simulink model "Sub_SC_G_based_221015"  (R2022b)
settings: Solver=VariableStepAuto  StartTime=0.0  StopTime=10.0  RelTol=1e-3
undefined symbols (not defined in the file or in its folder): R_bal, SC_rc, SC_rv
libraries: spsCurrentMeasurementLib x2, spsSeriesRLCBranchLib x2, spsSupercapacitorLib x1
settings Model: Creator=xuupp  LastModifiedBy=xuupp

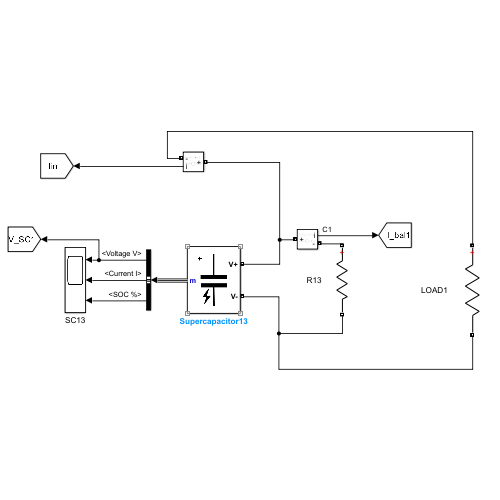
[thumbnail: Simulink's stored preview of the top-level diagram]
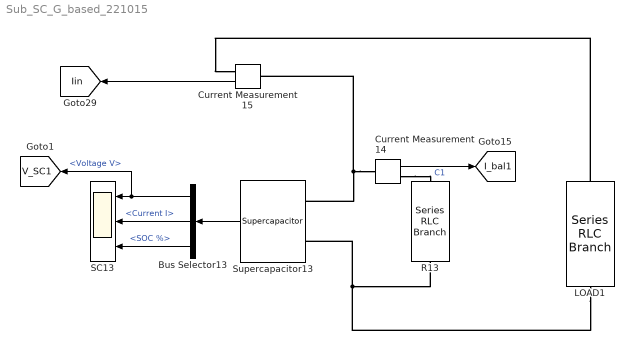
== system Sub_SC_G_based_221015 ==
  Bus Selector13 : BusSelector  OutputSignals=Voltage V,Current I,SOC %
  Current Measurement14 : spsCurrentMeasurementLib/Current Measurement  PhasorSimulation=off  OutputType=Complex  PSBequivalent=0
  Current Measurement15 : spsCurrentMeasurementLib/Current Measurement  PhasorSimulation=off  OutputType=Complex  PSBequivalent=0
  LOAD1 : spsSeriesRLCBranchLib/Series RLC Branch  LConnTagsString=__new0  RConnTagsString=__new0  BranchType=R  Resistance=10  Inductance=1e-3  SetiL0=off  InitialCurrent=0  Capacitance=1e-5  Setx0=on  InitialVoltage=0  Measurements=Branch voltage and current
  R13 : spsSeriesRLCBranchLib/Series RLC Branch  LConnTagsString=__new0  RConnTagsString=__new0  BranchType=R  Resistance=R_bal  Inductance=1e-3  SetiL0=off  InitialCurrent=0  Capacitance=54.3e-6  Setx0=on  InitialVoltage=160  Measurements=None
  SC13 : Scope  NumInputPorts=3
  Supercapacitor13 : spsSupercapacitorLib/Supercapacitor  C=SC_rc  Rdc=8.9e-3  Voltage=SC_rv  Ns=50  Np=16  Vinit=SC_iv  Temp=25  PresetModel=off  EstParam=off  Nc=1  r=1e-9  epsilon=6.0208e-10  Ich=10  Vstern="[0.161  2.7  7.8]"  Self_dis=off  Ioc=10  Vself="[48  47.8  47.06  44.65]"  demandeplot=off  I="[10  20 100  500]"  Units=sec  Vmax=0  If=0  deltaV=0  alpha=0  sec=0
      settings: LibrarySourceBlock=sps_lib/Sources/Supercapacitor
  tag scope: I_bal1=global, Iin=global, V_SC1=global
  wires:
  Supercapacitor13/1 -> Bus Selector13/1
  Bus Selector13/3 -> SC13/3  "<SOC %>"
  Bus Selector13/2 -> SC13/2  "<Current I>"
  Bus Selector13/1 -> SC13/1, [V_SC1]  "<Voltage V>"
  Current Measurement15/1 -> [Iin]
  Current Measurement14/1 -> [I_bal1]  "C1"
  connections:
  Current Measurement14/LConn1 -- Current Measurement15/LConn1 -- Supercapacitor13/LConn1
  Supercapacitor13/LConn2 -- R13/RConn1 -- LOAD1/RConn1
  LOAD1/LConn1 -- Current Measurement15/RConn1
  Current Measurement14/RConn1 -- R13/LConn1
